simulink library "PC_Simulator_Lib"  (Simulink 8.2)
settings: Solver=ode45  StartTime=0.0  StopTime=10.0  RelTol=1e-3
values from neighbouring files (symbols this model uses):
  data = [r1 r2 r3 r4 L1 L2 L3 L4]    [strasse_Bedatung_HNI_ITI.m]
  distSameLane = 60    [InitialisationsEnv.m]
  eng_speed = [0 60 120 180 240 300 360 420 480 540 600 660 ... (101 elements, 1x101)]    [engine_table.mat]    (also in motor_parameter_calc.m = omega)
  Heading_init = 0    [Start.m]
  inertiaLateral = 25*(radiusWheel)^2    (= 4.129024)    [Start.m]
  laneWidth = 3.6    [InitialisationsEnv.m]    (also in strasse_Bedatung_HNI_ITI.m)
  omega_engine = [0.000000 150.000000 500.000000 1000.000000 1500.000000 2000.000000 2500.000000 3000.000000 3500.000000 4000.000000 4500.000000 5000.000000 5500.000000 6000.000000]    [friction_tables.m]
  omega_max = 6000    [engine_table.mat]    (also in motor_parameter_calc.m)
  omega_wheel = [0 20 40 60 80 100 122 143.7 164]    [friction_tables.m]
  para_Fellow_8_Points = ADAS.Fellow_8_Points    [ADAS_parameters.m]
  position_start_x = [x1 x2 x3 x4 x5 x6 x7]    [strasse_Bedatung_HNI_ITI.m]
  position_start_y = [y1 y2 y3 y4 y5 y6 y7]    [strasse_Bedatung_HNI_ITI.m]
  rad3rdLine = 57.2    [InitialisationsEnv.m]    (also in strasse_Bedatung_HNI_ITI.m)
  radiusWheel = 16*2.54/100    (= 0.4064)    [Start.m]
  s_values = [S1 S2 S3 S4 S5 S6 S7]    [strasse_Bedatung_HNI_ITI.m]
  segmentLimits = [segment1EndThirdLine                   segment2EndThirdLine                   segment3EndThirdLine                   segment4EndThirdLine                   segment5EndThirdLine                   segment6EndThirdLine                   segment7EndThirdLine                   segment8EndThirdLine                   ]    [InitialisationsEnv.m]    (also in strasse_Bedatung_HNI_ITI.m)
  setPosT = [-1.8 -5.4 -1.8 -5.4 -1.8 -5.4 -1.8 -5.4 -1.8 -5.4]    [InitialisationsEnv.m]
  torque = [297.089227105 300.997600937 304.800343044 308.497453426 312.088932082 315.574779014 318.95499422 322.229577701 325.398529457 328.461849487 331.419537793 334.271594373 ... (101 elements, 1x101)]    [engine_table.mat]    (also in motor_parameter_calc.m = g)
  Torque_lost = [0.000000 -8.777780 -15.000000 -26.800000 -29.600000 -32.700000 -35.900000 -39.300000 -42.800000 -46.500000 -50.300000 -54.300000 -58.500000 -62.800000 ]*0.6    [friction_tables.m]
  Torque_lost_wheel = [0.8 0.8 0.75 0.7 0.4 0.3 0.2 0.07 0.07]*0.2    [friction_tables.m]
  X_init = 0    [Start.m]
  Y_init = 1.8    [Start.m]
  Z_init = 0    [Start.m]
undefined symbols (not defined in the file or in its folder): Acc_Pedal, ADAS, Brake_Pedal, Joystick, Newton, Para, Raphson, Standard_Devices, Steering_Wheel_Angle, UDP_Protocol
libraries: simulink x43, rtwinlib x7, dspnetwork x2, simulink_extras x1, vrlib x1
(part 13 of 13)

== matlab function ADAS/Sensors_ADAS/Front_Mid_Range_Radar_Sensor/First_STage_Coordinate_Transformation/Triangles_2_Fellows_Coord_Transformation_Plus_Sphere_Filtering/MATLAB Function ==
  data: Triangles_Points_Glob input double; Positon_Fellows input double; Oriantation_Fellows input double; Position_VUT input double; Upper_Triangles output double; Central_Triangles output double; Lower_Triangles output double; para_num_fellow parameter double; Inside_Sphere output double; para_filter_radius parameter double
function [Upper_Triangles,Central_Triangles,Lower_Triangles,Inside_Sphere] = fcn(Triangles_Points_Glob,Positon_Fellows,Oriantation_Fellows,Position_VUT,para_num_fellow,para_filter_radius)
%%
Upper_Triangle=zeros(para_num_fellow,9);
Central_Triangle=zeros(para_num_fellow,9);
Lower_Triangle=zeros(para_num_fellow,9);
is_inside=zeros(para_num_fellow,1);
for i=0:para_num_fellow-1
D=sqrt((Position_VUT(1)-Positon_Fellows(i*3+1))^2+(Position_VUT(2)-Positon_Fellows(i*3+2))^2+(Position_VUT(3)-Positon_Fellows(i*3+3))^2);   
if D<para_filter_radius
    is_inside(i+1)=1;
end
end
% pass inputs and calculate the transformation matrix
for i=0:para_num_fellow-1
    if is_inside(i+1)==1
roll=Oriantation_Fellows(i*3+1);
pitch=Oriantation_Fellows(i*3+2);
yaw=Oriantation_Fellows(i*3+3);
Trans_Global2Local=[ cos(pitch)*cos(yaw) cos(yaw)*sin(pitch)*sin(roll) - cos(roll)*sin(yaw) sin(roll)*sin(yaw) + cos(roll)*cos(yaw)*sin(pitch);
cos(pitch)*sin(yaw) cos(roll)*cos(yaw) + sin(pitch)*sin(roll)*sin(yaw) cos(roll)*sin(pitch)*sin(yaw) - cos(yaw)*sin(roll);
         -sin(pitch)                               cos(pitch)*sin(roll)                               cos(pitch)*cos(roll)]';
     
%%
%Transform each single point and save them in variables
Apex=Trans_Global2Local*([Triangles_Points_Glob(1) ; Triangles_Points_Glob(2) ; Triangles_Points_Glob(3)]-[Positon_Fellows(i*3+1);Positon_Fellows(i*3+2);Positon_Fellows(i*3+3)]);
Centeral_Triangle_LeftPoint=Trans_Global2Local*([Triangles_Points_Glob(4) ; Triangles_Points_Glob(5) ; Triangles_Points_Glob(6)]-[Positon_Fellows(i*3+1);Positon_Fellows(i*3+2);Positon_Fellows(i*3+3)]);
Centeral_Triangle_RightPoint=Trans_Global2Local*([Triangles_Points_Glob(7) ; Triangles_Points_Glob(8) ; Triangles_Points_Glob(9)]-[Positon_Fellows(i*3+1);Positon_Fellows(i*3+2);Positon_Fellows(i*3+3)]);
Upper_Triangle_LeftPoint=Trans_Global2Local*([Triangles_Points_Glob(10) ; Triangles_Points_Glob(11) ; Triangles_Points_Glob(12)]-[Positon_Fellows(i*3+1);Positon_Fellows(i*3+2);Positon_Fellows(i*3+3)]);
Upper_Triangle_RightPoint=Trans_Global2Local*([Triangles_Points_Glob(13) ; Triangles_Points_Glob(14) ; Triangles_Points_Glob(15)]-[Positon_Fellows(i*3+1);Positon_Fellows(i*3+2);Positon_Fellows(i*3+3)]);
Lower_Triangle_LeftPoint=Trans_Global2Local*([Triangles_Points_Glob(16) ; Triangles_Points_Glob(17) ; Triangles_Points_Glob(18)]-[Positon_Fellows(i*3+1);Positon_Fellows(i*3+2);Positon_Fellows(i*3+3)]);
Lower_Triangle_RightPoint=Trans_Global2Local*([Triangles_Points_Glob(19) ; Triangles_Points_Glob(20) ; Triangles_Points_Glob(21)]-[Positon_Fellows(i*3+1);Positon_Fellows(i*3+2);Positon_Fellows(i*3+3)]);
Upper_Triangle(i+1,:)=[Apex ; Upper_Triangle_LeftPoint ; Upper_Triangle_RightPoint];
Central_Triangle(i+1,:)=[Apex ; Centeral_Triangle_LeftPoint ; Centeral_Triangle_RightPoint];
Lower_Triangle(i+1,:)=[Apex ; Lower_Triangle_LeftPoint ; Lower_Triangle_RightPoint];
    end
end
%%
%pass the output
Upper_Triangles=reshape(Upper_Triangle.',1,[])';
Central_Triangles=reshape(Central_Triangle.',1,[])';
Lower_Triangles=reshape(Lower_Triangle.',1,[])';
Inside_Sphere=is_inside;

== matlab function ADAS/Sensors_ADAS/convert_xy_2_st1/Embedded MATLAB Function ==
  data: data input double; position_start_x input double; position_start_y input double; s_values input double; Positon_of_detected_Points input double; z output double; psi output double; mue output double; s output double; t output double; para_num_fellow parameter double
function [z,psi,mue,s,t] = fcn(data,position_start_x,position_start_y,s_values,Positon_of_detected_Points,para_num_fellow)

x=zeros(para_num_fellow,2);
y=zeros(para_num_fellow,2);
t_array=zeros(para_num_fellow,2);
for j=1:2
for i=1:para_num_fellow
    x(i,j)=Positon_of_detected_Points(i,1,j);
    y(i,j)=Positon_of_detected_Points(i,2,j);
end
end
breite=14.4;
margin=5;
for j=1:2
for i=1:para_num_fellow
if x(i,j)>=0 && x(i,j)<position_start_x(1) && y(i,j)>=-(breite/2+margin) && y(i,j)<=(breite/2+margin)                                               %S1
    s=x(i,j);
    t_array(i,j)=y(i,j);
    psi=0;
else if x(i,j)>=position_start_x(1) && x(i,j)<(position_start_x(2)+breite/2+margin) && y(i,j)>=-(breite/2+margin) && y(i,j)<=position_start_y(2)    %S2
        phi=atan((x(i,j)-position_start_x(1))/(position_start_y(2)-y(i,j)));
        r=sqrt((x(i,j)-position_start_x(1))^2 + (position_start_y(2)-y(i,j))^2);
        s=data(1)*phi+s_values(1);
        t_array(i,j)=data(1)-r;
        psi=phi;
        
else if x(i,j)>=(position_start_x(2)-breite/2-margin) && x(i,j)<=(position_start_x(2)+breite/2+margin) && y(i,j)>position_start_y(2) && y(i,j)<position_start_y(3)  %S3
        s=s_values(2)+(y(i,j)-position_start_y(2));
        t_array(i,j)=position_start_x(2)-x(i,j);
        psi=pi/2;
        
else if  x(i,j)<=(position_start_x(3)+breite/2+margin) && x(i,j)>=(position_start_x(4)) && y(i,j)>=position_start_y(3) && y(i,j)<=(position_start_y(4)+breite/2+margin)   %S4
        phi=atan((y(i,j)-position_start_y(3))/(x(i,j)-position_start_x(4)));
        r=sqrt((y(i,j)-position_start_y(3))^2+(x(i,j)-position_start_x(4))^2);
        s=s_values(3)+data(2)*phi;
        t_array(i,j)=data(2)-r;
        psi=pi/2+phi;
        
else if x(i,j)<position_start_x(4) && x(i,j)>position_start_x(5) && y(i,j)>=(position_start_y(4)-breite/2-margin) && y(i,j)<(position_start_y(4)+breite/2+margin)   %S5
        s=s_values(4)+(position_start_x(4)-x(i,j));
        t_array(i,j)=position_start_y(4)-y(i,j);
        psi=pi;
        
else if x(i,j)<=position_start_x(5) && x(i,j)>=(position_start_x(6)-breite/2-margin) && y(i,j)>=position_start_y(6) && y(i,j)<=(position_start_y(5)+breite/2+margin)   %S6
        phi=atan(-x(i,j)/(y(i,j)-position_start_y(6)));
        r=sqrt((x(i,j))^2+(y(i,j)-position_start_y(6))^2);
        s=s_values(5)+data(3)*phi;
        t_array(i,j)=data(3)-r;
        psi=pi+phi;
        
else if x(i,j)>=(position_start_x(6)-breite/2-margin) && x(i,j)<=(position_start_x(6)+breite/2+margin) && y(i,j)>position_start_y(7) && y(i,j)<position_start_y(6)   %S7
        s=s_values(6)+(position_start_y(6)-y(i,j));
        t_array(i,j)=x(i,j)-position_start_x(6);
        psi=3*pi/2;
        
else if x(i,j)>=(position_start_x(7)-breite/2-margin) && x(i,j)<0 && y(i,j)>=(-breite/2-margin) && y(i,j)<=position_start_y(7)   %S8
        phi=atan((position_start_y(7)-y(i,j))/(-x(i,j)));
        r=sqrt((position_start_y(7)-y(i,j))^2+(x(i,j))^2);
        s=s_values(7)+data(4)*phi;
        t_array(i,j)=data(4)-r;
        psi=3*pi/2+phi;     
        

     else
         s=0;
         t_array(i,j)=0;
         psi=0;

    end
    end
    end
    end
    end
    end
    end
end
end
end
t=t_array;    
z=0;
mue=1;

== matlab function ADAS/Sensors_ADAS/Front_Long_Range_Radar_Sensor/First_STage_Coordinate_Transformation/Triangles_2_Fellows_Coord_Transformation_Plus_Sphere_Filtering/MATLAB Function ==
  data: Triangles_Points_Glob input double; Positon_Fellows input double; Oriantation_Fellows input double; Position_VUT input double; Upper_Triangles output double; Central_Triangles output double; Lower_Triangles output double; para_num_fellow parameter double; Inside_Sphere output double; para_filter_radius parameter double
function [Upper_Triangles,Central_Triangles,Lower_Triangles,Inside_Sphere] = fcn(Triangles_Points_Glob,Positon_Fellows,Oriantation_Fellows,Position_VUT,para_num_fellow,para_filter_radius)
%%
Upper_Triangle=zeros(para_num_fellow,9);
Central_Triangle=zeros(para_num_fellow,9);
Lower_Triangle=zeros(para_num_fellow,9);
is_inside=zeros(para_num_fellow,1);
for i=0:para_num_fellow-1
D=sqrt((Position_VUT(1)-Positon_Fellows(i*3+1))^2+(Position_VUT(2)-Positon_Fellows(i*3+2))^2+(Position_VUT(3)-Positon_Fellows(i*3+3))^2);   
if D<para_filter_radius
    is_inside(i+1)=1;
end
end
% pass inputs and calculate the transformation matrix
for i=0:para_num_fellow-1
    if is_inside(i+1)==1
roll=Oriantation_Fellows(i*3+1);
pitch=Oriantation_Fellows(i*3+2);
yaw=Oriantation_Fellows(i*3+3);
Trans_Global2Local=[ cos(pitch)*cos(yaw) cos(yaw)*sin(pitch)*sin(roll) - cos(roll)*sin(yaw) sin(roll)*sin(yaw) + cos(roll)*cos(yaw)*sin(pitch);
cos(pitch)*sin(yaw) cos(roll)*cos(yaw) + sin(pitch)*sin(roll)*sin(yaw) cos(roll)*sin(pitch)*sin(yaw) - cos(yaw)*sin(roll);
         -sin(pitch)                               cos(pitch)*sin(roll)                               cos(pitch)*cos(roll)]';
     
%%
%Transform each single point and save them in variables
Apex=Trans_Global2Local*([Triangles_Points_Glob(1) ; Triangles_Points_Glob(2) ; Triangles_Points_Glob(3)]-[Positon_Fellows(i*3+1);Positon_Fellows(i*3+2);Positon_Fellows(i*3+3)]);
Centeral_Triangle_LeftPoint=Trans_Global2Local*([Triangles_Points_Glob(4) ; Triangles_Points_Glob(5) ; Triangles_Points_Glob(6)]-[Positon_Fellows(i*3+1);Positon_Fellows(i*3+2);Positon_Fellows(i*3+3)]);
Centeral_Triangle_RightPoint=Trans_Global2Local*([Triangles_Points_Glob(7) ; Triangles_Points_Glob(8) ; Triangles_Points_Glob(9)]-[Positon_Fellows(i*3+1);Positon_Fellows(i*3+2);Positon_Fellows(i*3+3)]);
Upper_Triangle_LeftPoint=Trans_Global2Local*([Triangles_Points_Glob(10) ; Triangles_Points_Glob(11) ; Triangles_Points_Glob(12)]-[Positon_Fellows(i*3+1);Positon_Fellows(i*3+2);Positon_Fellows(i*3+3)]);
Upper_Triangle_RightPoint=Trans_Global2Local*([Triangles_Points_Glob(13) ; Triangles_Points_Glob(14) ; Triangles_Points_Glob(15)]-[Positon_Fellows(i*3+1);Positon_Fellows(i*3+2);Positon_Fellows(i*3+3)]);
Lower_Triangle_LeftPoint=Trans_Global2Local*([Triangles_Points_Glob(16) ; Triangles_Points_Glob(17) ; Triangles_Points_Glob(18)]-[Positon_Fellows(i*3+1);Positon_Fellows(i*3+2);Positon_Fellows(i*3+3)]);
Lower_Triangle_RightPoint=Trans_Global2Local*([Triangles_Points_Glob(19) ; Triangles_Points_Glob(20) ; Triangles_Points_Glob(21)]-[Positon_Fellows(i*3+1);Positon_Fellows(i*3+2);Positon_Fellows(i*3+3)]);
Upper_Triangle(i+1,:)=[Apex ; Upper_Triangle_LeftPoint ; Upper_Triangle_RightPoint];
Central_Triangle(i+1,:)=[Apex ; Centeral_Triangle_LeftPoint ; Centeral_Triangle_RightPoint];
Lower_Triangle(i+1,:)=[Apex ; Lower_Triangle_LeftPoint ; Lower_Triangle_RightPoint];
    end
end
%%
%pass the output
Upper_Triangles=reshape(Upper_Triangle.',1,[])';
Central_Triangles=reshape(Central_Triangle.',1,[])';
Lower_Triangles=reshape(Lower_Triangle.',1,[])';
Inside_Sphere=is_inside;

== matlab function Environment/Environment_Model/Road model/st_xy ==
  data: x output double; s input double; t input double; y output double; z output double; headingAngle output double; segmentLimits input double; laneWidth input double; rad3rdLine input double
function [x, y, z, headingAngle]   = st_xy(s, t, segmentLimits, laneWidth, rad3rdLine)
%% Description
% This function transforms the (s,t) points of the road to (x,y) points
% From local coordinate system to global coordinate system
% s,t: s,t points of the local coordinate system in meters
% segmentLimits: Limits, i.e. ends, of road segments in meters
% laneWidth: The width of the lane in meter
% rad3rdLine: Radius of the third line, i.e lane marking, in meter  
% x,y: x,y points of the global coordinate system in meters
% headingAngle: Heading angle of the road at a specific road segment
% curvature: Curvature of the road at a specific road segment
% segmentNr: Segment number of a specific (s,t) point on the road
%% Simple schematic for a slice of the road
%     |          |         |          |          |
% FirstLine SecondLine ThirdLine FourthLine FifthLine 
%        Lane 2     Lane 1    Lane -1    Lane -2
%% Simple schematic for the road shape
%  _____________________
% (                     )
% |                     |
% |                     |
% |                     |
% (_____________________)

%% Initialise the outputs (Assign default values)
% Initialise x with zero
x = zeros(1,length(s)); 
% Initialise y with zero
y = zeros(1,length(s));
% Initialise z with zero
z = zeros(1,length(s));
% Initialise headingAngle with zero
headingAngle = zeros(1,length(s));

% Go through all traffic vehicles
for vehicCount = 1 : length(s)
%% Check (s,t) point against all segments
%% Check if the point is in the 1st road segment (Straight line)
if(s(vehicCount)>=0)&&(s(vehicCount)<segmentLimits(1))  
    % Calculate x component
    x(vehicCount) = s(vehicCount);
    % Calculate y component
    y(vehicCount) = t(vehicCount);
    % Calculate z value
    z(vehicCount) = 0;
    % Calculate heading angle
    headingAngle(vehicCount) = 0;
%% Check if the point is in the 2nd road segment
elseif(s(vehicCount)>=segmentLimits(1)) && (s(vehicCount)<segmentLimits(2)) 
    % Calculate x component
    x(vehicCount) = (rad3rdLine-t(vehicCount))*sin((s(vehicCount)-segmentLimits(1))/rad3rdLine) + 600;
    % Calculate y component
    y(vehicCount) = rad3rdLine - (rad3rdLine-t(vehicCount))*cos((s(vehicCount)-segmentLimits(1))/rad3rdLine);
    % Calculate z value
    z(vehicCount) = 0;
    % Calculate heading angle
    headingAngle(vehicCount) = (180/pi)*(s(vehicCount)-600)/rad3rdLine;
%% Check if the point is in the 3rd road segment  
elseif(s(vehicCount)>=segmentLimits(2)) && (s(vehicCount)<segmentLimits(3))
    % Calculate x component
    x(vehicCount) = -t(vehicCount) + 600 + rad3rdLine;
    % Calculate y component
    y(vehicCount) = (s(vehicCount)-segmentLimits(2)) + rad3rdLine;
    % Calculate z value
    z(vehicCount) = 0;
    % Calculate heading angle
    headingAngle(vehicCount) = 90;
%% Check if the point is in the 4th road segment
elseif(s(vehicCount)>=segmentLimits(3)) && (s(vehicCount)<segmentLimits(4))
    % Calculate x component
    x(vehicCount) = (rad3rdLine-t(vehicCount))*cos((s(vehicCount)-segmentLimits(3))/rad3rdLine) - rad3rdLine + 600 + rad3rdLine;
    % Calculate y component
    y(vehicCount) = (rad3rdLine-t(vehicCount))*sin((s(vehicCount)-segmentLimits(3))/rad3rdLine) + 300 + rad3rdLine;
    % Calculate z value
    z(vehicCount) = 0;
    % Calculate heading angle
    headingAngle(vehicCount) = ((180/pi)*(s(vehicCount)-(600+89.8857+300))/rad3rdLine) + 90;
%% Check if the point is in the 5th road segment
elseif(s(vehicCount)>=segmentLimits(4))&&(s(vehicCount)<segmentLimits(5))
    % Calculate x component
    x(vehicCount) = -(s(vehicCount)-segmentLimits(4)) + 600;
    % Calculate y component
    y(vehicCount) = -t(vehicCount) + (4*laneWidth) + 50 + 300 + 50;
    % Calculate z value
    z(vehicCount) = 0;
    % Calculate heading angle
    headingAngle(vehicCount) = 180;
%% Check if the point is in the 6th road segment  
elseif(s(vehicCount)>=segmentLimits(5))&&(s(vehicCount)<segmentLimits(6))
    % Calculate x component
    x(vehicCount) = -(rad3rdLine-t(vehicCount))*sin((s(vehicCount)-segmentLimits(5))/rad3rdLine);
    % Calculate y component
    y(vehicCount) = (rad3rdLine-t(vehicCount))*cos((s(vehicCount)-segmentLimits(5))/rad3rdLine)- rad3rdLine + (4*laneWidth) + 50 + 300 + 50;
    % Calculate z value
    z(vehicCount) = 0;
    % Calculate heading angle
    headingAngle(vehicCount) = ((180/pi)*(s(vehicCount)-(600+89.8857+300+89.8857+600))/rad3rdLine) + 180;
%% Check if the point is in the 7th road segment 
elseif(s(vehicCount)>=segmentLimits(6))&&(s(vehicCount)<segmentLimits(7))
    % Calculate x component
    x(vehicCount) = t(vehicCount)- 50 - 3.6 - 3.6;
    % Calculate y component
    y(vehicCount) = -(s(vehicCount)-segmentLimits(6)) + (2*laneWidth) + 300 + 50;
    % Calculate z value
    z(vehicCount) = 0;
    % Calculate heading angle
    headingAngle(vehicCount) = 270;
%% Check if the point is in the 8th road segment 
elseif(s(vehicCount)>=segmentLimits(7))&&(s(vehicCount)<segmentLimits(8))
    % Calculate x component
    x(vehicCount) = rad3rdLine-(rad3rdLine-t(vehicCount))*cos((s(vehicCount)-segmentLimits(7))/rad3rdLine) - rad3rdLine;
    % Calculate y component
    y(vehicCount) = -(rad3rdLine-t(vehicCount))*sin((s(vehicCount)-segmentLimits(7))/rad3rdLine) + rad3rdLine; 
    % Calculate z value
    z(vehicCount) = 0;
    % Calculate heading angle
    headingAngle(vehicCount) = ((180/pi)*(s(vehicCount)-(600+89.8857+300+89.8857+600+89.8857+300))/rad3rdLine) + 270;
end
end

end

== matlab function Environment/Maping_Input /Strasse_xy/Embedded MATLAB Function ==
  data: data input double; position_start_x input double; position_start_y input double; s_values input double; x input double; y input double; z output double; psi output double; mue output double; s output double; t output double
function [z,psi,mue,s,t] = fcn(data,position_start_x,position_start_y,s_values,x,y)


breite=14.4;
margin=3;

if x>=0 && x<position_start_x(1) && y>=-(breite/2+margin) && y<=(breite/2+margin)                                               %S1
    s=x;
    t=y;
    psi=0;
else if x>=position_start_x(1) && x<(position_start_x(2)+breite/2+margin) && y>=-(breite/2+margin) && y<=position_start_y(2)    %S2
        phi=atan((x-position_start_x(1))/(position_start_y(2)-y));
        r=sqrt((x-position_start_x(1))^2 + (position_start_y(2)-y)^2);
        s=data(1)*phi+s_values(1);
        t=data(1)-r;
        psi=phi;
        
else if x>=(position_start_x(2)-breite/2-margin) && x<=(position_start_x(2)+breite/2+margin) && y>position_start_y(2) && y<position_start_y(3)  %S3
        s=s_values(2)+(y-position_start_y(2));
        t=position_start_x(2)-x;
        psi=pi/2;
        
else if  x<=(position_start_x(3)+breite/2+margin) && x>=(position_start_x(4)) && y>=position_start_y(3) && y<=(position_start_y(4)+breite/2+margin)   %S4
        phi=atan((y-position_start_y(3))/(x-position_start_x(4)));
        r=sqrt((y-position_start_y(3))^2+(x-position_start_x(4))^2);
        s=s_values(3)+data(2)*phi;
        t=data(2)-r;
        psi=pi/2+phi;
        
else if x<position_start_x(4) && x>position_start_x(5) && y>=(position_start_y(4)-breite/2-margin) && y<(position_start_y(4)+breite/2+margin)   %S5
        s=s_values(4)+(position_start_x(4)-x);
        t=position_start_y(4)-y;
        psi=pi;
        
else if x<=position_start_x(5) && x>=(position_start_x(6)-breite/2-margin) && y>=position_start_y(6) && y<=(position_start_y(5)+breite/2+margin)   %S6
        phi=atan(-x/(y-position_start_y(6)));
        r=sqrt((x)^2+(y-position_start_y(6))^2);
        s=s_values(5)+data(3)*phi;
        t=data(3)-r;
        psi=pi+phi;
        
else if x>=(position_start_x(6)-breite/2-margin) && x<=(position_start_x(6)+breite/2+margin) && y>position_start_y(7) && y<position_start_y(6)   %S7
        s=s_values(6)+(position_start_y(6)-y);
        t=x-position_start_x(6);
        psi=3*pi/2;
        
else if x>=(position_start_x(7)-breite/2-margin) && x<0 && y>=(-breite/2-margin) && y<=position_start_y(7)   %S8
        phi=atan((position_start_y(7)-y)/(-x));
        r=sqrt((position_start_y(7)-y)^2+(x)^2);
        s=s_values(7)+data(4)*phi;
        t=data(4)-r;
        psi=3*pi/2+phi;

        
        
        %%% from here will be terminated
% else if x>position_start_x(8) && x<position_start_x(9) && y>=(position_start_y(8)-breite/2-1)&& y<=(position_start_y(8)+breite/2+1)   %S9
%         s=s_values(8)+(x-position_start_x(8));
%         t=y-position_start_y(8);
%         psi=psi_flag;
%         
% else if x>=position_start_x(9) && x<=(position_start_x(10)+breite/2+1) && y>=(position_start_y(9)-breite/2-1)&& y<=position_start_y(10)  %S10
%         phi=atan((x-position_start_x(9))/(position_start_y(10)-y));
%         r=sqrt((x-position_start_x(9))^2+(position_start_y(10)-y)^2);
%         s=s_values(9)+phi*data(5);
%         t=data(5)-r;
%         psi=phi;
%         
% else if x>=(position_start_x(10)-breite/2-1) && x<=(position_start_x(10)+breite/2+1) && y>position_start_y(10)&& y<position_start_y(11)  %S11
%         
%         s=s_values(10)+(y-position_start_y(10));
%         t=position_start_x(10)-x;
%         psi=psi_flag;
%         
% else if x>=position_start_x(12) && x<=(position_start_x(11)+breite/2+1) && y>=position_start_y(11)&& y<=(position_start_y(12)+breite/2+1)  %S12
%         phi=atan((y-position_start_y(11))/(x-position_start_x(12)));
%         r=sqrt((y-position_start_y(11))^2+(x-position_start_x(12))^2);
%         s=s_values(11)+phi*data(6);
%         t=data(6)-r;
%         psi=pi/2+phi;
%         
% else if x>position_start_x(13) && x<position_start_x(12)&& y>=(position_start_y(12)-breite/2-1)&& y<=(position_start_y(12)+breite/2+1)  %S13
%         s=s_values(12)+(position_start_x(12)-x);
%         t=position_start_y(12)-y;
%         psi=psi_flag;
%         
% else if x>=(position_start_x(14)-breite/2-1) && x<=position_start_x(13)&& y>=position_start_y(14)&& y<=(position_start_y(13)+breite/2+1)  %S14
%         phi=atan((position_start_x(13)-x)/(y-position_start_y(14)));
%         r=sqrt((position_start_x(13)-x)^2+(y-position_start_y(14))^2);
%         s=s_values(13)+phi*data(7);
%         t=data(7)-r;
%         psi=pi+phi;
%         
% else if x>(position_start_x(14)-breite/2-1) && x<=(position_start_x(14)+breite/2+1)&& y>position_start_y(15)&& y<position_start_y(14)  %S15
%             s=s_values(14)+(position_start_y(14)-y);
%             t=x-position_start_x(14);
%             psi=psi_flag;
%             
% else if x>=(position_start_x(15)-breite/2-1) && x<=position_start_x(16)&& y>=(position_start_y(16)-breite/2-1)&& y<=position_start_y(15)  %S16
%         phi=atan((position_start_y(15)-y)/(position_start_x(16)-x));
%         r=sqrt((position_start_y(15)-y)^2+(position_start_x(16)-x)^2);
%         s=s_values(15)+phi*data(8);
%         t=data(8)-r;
%         psi=3*pi/2+phi;
%         
% else if x>position_start_x(16) && x<0 && y>-breite/2-1 && y< breite/2+1  %S17
%         s=s_values(16)+(x-position_start_x(16));
%         t=y-position_start_y(16);
%         psi=psi_flag;
     else
         s=0;
         t=0;
         psi=0;
%     end
%     end
%     end
%     end
%     end
%     end
%     end
%     end
%     end
%      end
    end
    end
    end
    end
    end
    end
    end
end
    
z=0;
mue=1;

== matlab function Comunication_with_visualisation_normal_mode/Embedded MATLAB Function ==
  data: u input double; y output double
function y = fcn(u)
%#eml

y = typecast(u,'uint8');

== matlab function Comunication_with_visualisation_normal_mode_new_Version/Embedded MATLAB Function ==
  data: u input double; y output double
function y = fcn(u)
%#eml

y = typecast(u,'uint8');

== matlab function Comunication_with_visualisation_Realtime_new_version/Embedded MATLAB Function ==
  data: u input double; y output double
function y = fcn(u)
%#eml

y = typecast(u,'uint8');

== stateflow chart ADAS/Unser_Interface_ADAS/Emergency_Steering/Emergency_steer_HMI_model ==
  state On
    en:
    State=1;
  state Off
    en:
    State=0;
  On -> Off : Button
  Off -> On : Button[Enabled_Systems==0]
  (default) -> Off
  data: State output double; Enabled_Systems input double
  events: Update input EITHER_EDGE_EVENT; Button input RISING_EDGE_EVENT

== stateflow chart ADAS/Unser_Interface_ADAS/Pilotiertes_Fahren/Pilotiertes_fahren_HMI_model ==
  state On
    en:
    State=1;
  state Off
    en:
    State=0;
  On -> Off [order 2] : [ Gearbox_State!=1 || Brake_Pedal_User>Brake_Pedal_ACC || Gas_Pedal_User>Gas_Pedal_ACC ]
  On -> Off [order 1] : Button
  Off -> On : Button[Enabled_Systems==0 && Gearbox_State==1 ]
  (default) -> Off
  data: State output double; Enabled_Systems input double; Gearbox_State input double; Gas_Pedal_User input double; Brake_Pedal_User input double; Gas_Pedal_ACC input double; Brake_Pedal_ACC input double
  events: Update input EITHER_EDGE_EVENT; Button input RISING_EDGE_EVENT

== matlab function ADAS/Sensors_ADAS/Front_Long_Range_Radar_Sensor/First_STage_Coordinate_Transformation/Radar_Triangles_Transformation_From_Local2Global/Coord_Transformatin_Rotation ==
  data: roll input double; Trans_Local2Global output double; pitch input double; yaw input double
function Trans_Local2Global  = fcn(roll, pitch, yaw)


Trans_Local2Global=[ cos(pitch)*cos(yaw) cos(yaw)*sin(pitch)*sin(roll) - cos(roll)*sin(yaw) sin(roll)*sin(yaw) + cos(roll)*cos(yaw)*sin(pitch);
cos(pitch)*sin(yaw) cos(roll)*cos(yaw) + sin(pitch)*sin(roll)*sin(yaw) cos(roll)*sin(pitch)*sin(yaw) - cos(yaw)*sin(roll);
         -sin(pitch)                               cos(pitch)*sin(roll)                               cos(pitch)*cos(roll)];

== matlab function Environment/Environment_Model/Senario manager ==
  data: actualPosT input double; mainCarPosS input double; mainCarPosT input double; allowedDistS input double; desiredPosT output double; desiredPosS output double; ADAS input double; desiredYaw output double
function [desiredPosT, desiredPosS, desiredYaw]  = Scenarios(actualPosT, mainCarPosS, mainCarPosT, allowedDistS, ADAS)

desiredPosS = 0;
desiredPosT = -9;
desiredYaw = 0;


if actualPosT == -9
%     desiredPosT =   - 0.75 + mainCarPosT;
        desiredPosT =   - 1.8365 -5.4;

    %- 1.8365 +
end

%% If no ADAS is activated
if ADAS == 1      
    if mainCarPosS >= 0 && mainCarPosS <= 600
        desiredPosS = 380;
        if (desiredPosS - mainCarPosS <= allowedDistS)
    
            desiredYaw = 90;
%             desiredPosT =  - 0.75 + mainCarPosT;
            desiredPosT =  - 1.8365 -5.4;
        end     
    elseif mainCarPosS >= 689 && mainCarPosS <= 989
        desiredPosS = 900;
        if (desiredPosS - mainCarPosS <= allowedDistS)

            desiredYaw = 180;
%             desiredPosT =  - 0.75 + mainCarPosT;
            desiredPosT =  - 1.8365 -5.4;
        end      
    elseif mainCarPosS >= 1079 && mainCarPosS <= 1679
        desiredPosS = 1379;
        if (desiredPosS - mainCarPosS <= allowedDistS)
  
            desiredYaw = 270;
            %             desiredPosT =  - 0.75 + mainCarPosT;
            desiredPosT =  - 1.8365 -5.4;
        end        
    elseif mainCarPosS >= 1769 && mainCarPosS <= 2069
        desiredPosS = 1969;
        if (desiredPosS - mainCarPosS <= allowedDistS)

            desiredYaw = 360;
            %             desiredPosT =  - 0.75 + mainCarPosT;
            desiredPosT =  - 1.8365 -5.4;
        end      
    end  
end

== matlab function Environment/Environment_Model/Master driver/masterDriver ==
  data: desiredVelS output double; setVelS input double; setPosT input double; actualPosS input double; actualPosT input double; actualVelS input double; distSameLanes input double; mainCarPosS input double; desiredPosT output double; mainCarPosT input double; mainCarVelS input double; mainCarWidth input double
function [desiredVelS, desiredPosT] = masterDriver(setVelS, setPosT, actualPosS, actualPosT, actualVelS, distSameLanes, mainCarPosS, mainCarPosT, mainCarVelS, mainCarWidth)
% This function determines the behaviour of the traffic vehicles
%--------------------------------------------------------------------------
%% Inputs description
%--------------------
% setVelS: A vector of set s-velocities of all traffic vehicles [km/h]
% setPosT: A vector of set t-positions of all traffic vehicles [m]
% actualPosS: A vector of actual s-positions of all traffic vehicles [m]
% actualPosT: A vector of actual t-positions of all traffic vehicles [m]
% actualVelS: A vector of actual s-velocities of all traffic vehicles [m/s] 
% distSameLanes: Allowed distance between two vehicles in same lanes [m]
% mainCarPosS: Current poistion of the main vehicle [m] 
%--------------------------------------------------------------------------
%% Outputs description
%---------------------
% desiredVelS: A vector of desired s-velocities of all traffic vehicles [km/h]
% desiredPosT: A vector of desired t-positions of all traffic vehicles [m]
%--------------------------------------------------------------------------
%% Initialisation of outputs
%---------------------------
% Let the s-velocities of vehicles equal to the set s-velocities
desiredVelS = setVelS;
% Let the t-positions of vehicles equal to the set t-positions
desiredPosT = setPosT;
%--------------------------------------------------------------------------
%% Calculations
%----------------------
% Convert all actual s-velocities from [m/s] to [km/h]
actualVelS = actualVelS*(3.6);               
% %------------------------------------------------------------------------
% % Avoid collision of traffic vehicles with each other
% %-----------------------------------------
% % |x|-|-|-|
% % | |x|-|-|
% % | | |x|-|    Create a matrix of all traffic vehicles
% % | | | |x|
% Go through the matrix vertically 
for carCounterV = 1 : length(actualPosS)
    % Go through the matrix horizontally 
    for carCounterH = 1 : length(actualPosS)
        % If it is not a diagonal position of the matrix
        % And if it is not in the matrix mirror
        if carCounterH < carCounterV
            % Check if they are in the same lane
            if actualPosT(carCounterV) == actualPosT(carCounterH) 
                % Check if the allowed distance is exceeded
                if abs(actualPosS(carCounterV) - actualPosS(carCounterH)) <= distSameLanes
                    % Check which car is faster
                    if (actualVelS(carCounterV) > actualVelS(carCounterH)) && (actualPosS(carCounterV) < actualPosS(carCounterH))
                        desiredVelS(carCounterV) = actualVelS(carCounterH);                
                    % Check which car is faster    
                    elseif actualVelS(carCounterH) > actualVelS(carCounterV) && (actualPosS(carCounterH) < actualPosS(carCounterV))
                        desiredVelS(carCounterH) = actualVelS(carCounterV);                
                    end
                end   
            end 
        end
    end
end
% %------------------------------------------------------------------------
% % Avoid collision of traffic vehicles with main vehicle
% %-----------------------------------------
% Go through all traffic vehicles 
for trafVehic = 1 : length(actualPosS)
    % Check if the allowed distance is exceeded
    if abs(mainCarPosS - actualPosS(trafVehic)) < distSameLanes
        % Check if the traffic vehichle is behind the main vehicle
        if (actualPosS(trafVehic) < mainCarPosS) && (actualVelS(trafVehic) > mainCarVelS)
            % Check if the traffic vehicle is in the same lane of main car
            % Or if the main car is near the lane marking 
            if (actualPosT(trafVehic) == mainCarPosT) || (abs(actualPosT(trafVehic)-mainCarPosT) < (1.8+mainCarWidth/2))  
                desiredVelS(trafVehic) =  mainCarVelS;
            end    
        end      
    end
end





end
